simulink model "CorrienteH11"  (R2026a)
settings: Solver=FixedStepDiscrete  StopTime=1  FixedStep=1/2000  EnableMultiTasking=on
libraries: slpidlib x10
settings Model: SILPILModeSetting=veronly  ExtModeTrigDuration=10  Creator=Mutti  LastModifiedBy=Mutti
settings DataIOCC: SaveState=on  InspectSignalLogs=on
settings OptimizationCC: StrengthReduction=on  OptimizationPriority=Speed  UseRestrictQualifier=on
settings HardwareCC: ProdLargestAtomicInteger=Long  ProdLargestAtomicFloat=Double  ProdHWDeviceType=ARM Compatible->ARM Cortex-M
settings ModelReferenceCC: PropagateVarSize=During execution
settings RTWCC: SystemTargetFile=ert.tlc  GenCodeOnly=on  GenerateReport=on  BuildConfiguration=Faster Runs  IncludeHyperlinkInReport=on  LaunchReport=on  PortableWordSizes=on  CodeProfilingSaveOptions=AllData  TargetLang=C++  GenerateTraceInfo=on  GenerateTraceReport=on  GenerateTraceReportSl=on  GenerateTraceReportSf=on  GenerateTraceReportEml=on  GenerateWebview=on  GenerateCodeMetricsReport=on  GenerateCodeReplacementReport=on  Description=Embedded Coder
settings CodeAppCC: GenerateComments=off  SimulinkBlockComments=off
settings ERTTargetCC: ExtModeTransport=3.0  ExtModeStaticAllocSize=2048.0  RootIOFormat=Structure reference  TargetLangStandard=C++20 (ISO)  CodeReplacementLibrary=ARM Cortex-M  CodeInterfacePackaging=C++ class  SubcomponentCodeInterfacePackaging=C++ class  SupportNonFinite=off  SupportVariableSizeSignals=on

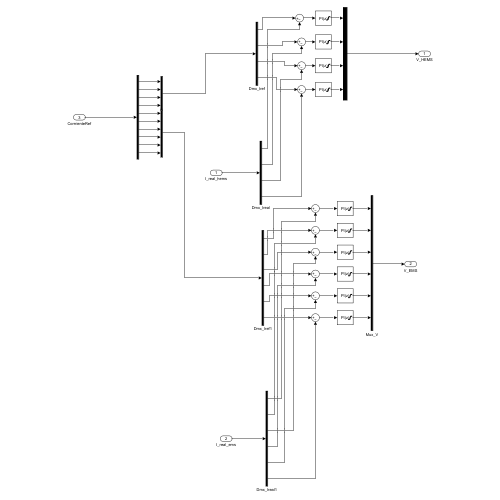
[thumbnail: Simulink's stored preview of the top-level diagram]
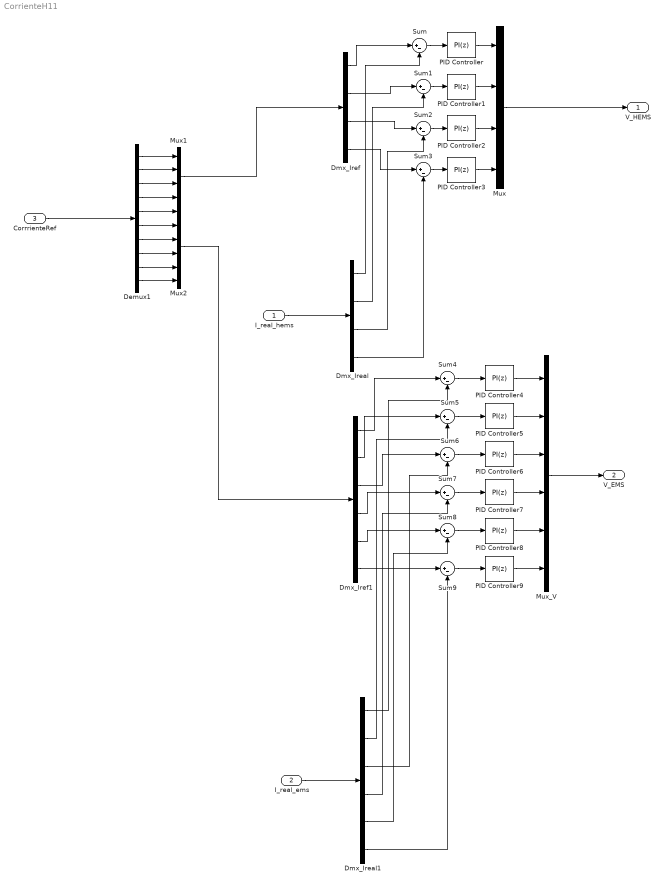
== system CorrienteH11 ==
  I_real_hems : Inport  OutDataTypeStr=double  PortDimensions=4  SampleTime=[0.00050000000000000001,0]
  I_real_ems : Inport  Port=2
  CorrrienteRef : Inport  Port=3
  Demux1 : Demux  Outputs=10
  Dmx_Ireal : Demux
  Dmx_Ireal1 : Demux  Outputs=6
  Dmx_Iref : Demux
  Dmx_Iref1 : Demux  Outputs=6
  Mux : Mux
  Mux1 : Mux
  Mux2 : Mux  Inputs=6
  Mux_V : Mux  Inputs=6
  PID Controller{,1..3} (4 alike) : slpidlib/PID Controller  Controller=PI  Form=Parallel  TimeDomain=Discrete-time  UseExternalTs=off  SampleTime=1/2000  IntegratorMethod=Trapezoidal  FilterMethod=Forward Euler  ControllerParametersSource=internal  P=4.54  I=500  UseKiTs=off  D=0  UseExternalDerivativeSource=off  N=100  UseFilter=on  TunerSelectOption=Transfer Function Based (PID Tuner App)  InitialConditionSource=internal  InitialConditionForIntegrator=0  InitialConditionForFilter=0  DifferentiatorICPrevScaledInput=0  ExternalReset=none  TrackingMode=off  Kt=1  LimitOutput=on  SatLimitsSource=internal  UpperSaturationLimit=350  LowerSaturationLimit=-350  LinearizeAsGain=on  AntiWindupMode=clamping  Kb=1  LimitIntegrator=on  UpperIntegratorSaturationLimit=350  LowerIntegratorSaturationLimit=-350  POutMin=[]  POutMax=[]  IOutMin=[]  IOutMax=[]  DOutMin=[]  DOutMax=[]  NOutMin=[]  NOutMax=[]  SumOutMin=[]  SumOutMax=[]  SaturationOutMin=[]  SaturationOutMax=[]  PParamMin=[]  PParamMax=[]  IParamMin=[]  IParamMax=[]  DParamMin=[]  DParamMax=[]  NParamMin=[]  NParamMax=[]  KbParamMin=[]  KbParamMax=[]  KtParamMin=[]  KtParamMax=[]  KbOutMin=[]  KbOutMax=[]  KtOutMin=[]  KtOutMax=[]  IntegratorOutMin=[]  IntegratorOutMax=[]  FilterOutMin=[]  FilterOutMax=[]  SumI1OutMin=[]  SumI1OutMax=[]  SumI2OutMin=[]  SumI2OutMax=[]  SumI3OutMin=[]  SumI3OutMax=[]  SumI4OutMin=[]  SumI4OutMax=[]  SumDOutMin=[]  SumDOutMax=[]  DifferentiatorOutMin=[]  DifferentiatorOutMax=[]  FilterDiffOutCoefMin=[]  FilterDiffOutCoefMax=[]  ReciprocalOutMin=[]  ReciprocalOutMax=[]  SumDenOutMin=[]  SumDenOutMax=[]  SumNumOutMin=[]  SumNumOutMax=[]  DivideOutMin=[]  DivideOutMax=[]  UdiffTsProdOutMin=[]  UdiffTsProdOutMax=[]  NTsProdOutMin=[]  NTsProdOutMax=[]  UintegralTsProdOutMin=[]  UintegralTsProdOutMax=[]  UngainTsProdOutMin=[]  UngainTsProdOutMax=[]  ClampingZeroOutDataTypeStr=Inherit: Inherit via back propagation  ClampingZeroOutMin=[]  ClampingZeroOutMax=[]  FilterDenConstantOutDataTypeStr=Inherit: Inherit via back propagation  FilterDenConstantOutMin=[]  FilterDenConstantOutMax=[]  PCopyOutDataTypeStr=Inherit: Inherit via back propagation  PCopyOutMin=[]  PCopyOutMax=[]  NCopyOutDataTypeStr=Inherit: Inherit via back propagation  NCopyOutMin=[]  NCopyOutMax=[]  IntegratorContinuousStateAttributes=''  IntegratorStateMustResolveToSignalObject=off  IntegratorRTWStateStorageClass=Auto  FilterContinuousStateAttributes=''  FilterStateMustResolveToSignalObject=off  FilterRTWStateStorageClass=Auto  ParallelPVariant=InternalParameters  IdealPVariant=Disabled  IVariant=InternalParameters  DVariant=Disabled  IntegratorVariant=Discrete  SatVariant=Enabled  AWVariant=DiscClampingParallel  PCopyVariant=Disabled  TRVariant=Disabled  FdbkBlocksVariant=Feedback  IdealPFdbkVariant=Passthrough  SatFdbkVariant=Passthrough  DerivativeFilterVariant=Disabled  NVariant=Disabled  NCopyVariant=Disabled_SignalSpec  FilterICVariant=Disabled  IntegratorICVariant=InternalICs  ExternalResetVariant=Disabled  TRSumVariant=Passthrough  SumFdbkVariant=Enabled  SumVariant=Sum_PI  TsampFilterVariant=InternalTs  TsampNgainVariant=Passthrough  TsampIntegralVariant=Disabled_SignalSpec  ExternalSaturationOutDataTypeStr=Inherit: Same as second input  DerivativeSourceVariant=Disabled  PreIntVariant=InternalPreInt
  PID Controller{4..9} (6 alike) : slpidlib/PID Controller  Controller=PI  Form=Parallel  TimeDomain=Discrete-time  UseExternalTs=off  SampleTime=1/2000  IntegratorMethod=Trapezoidal  FilterMethod=Forward Euler  ControllerParametersSource=internal  P=0.50390000000000001  I=70  UseKiTs=off  D=0  UseExternalDerivativeSource=off  N=100  UseFilter=on  TunerSelectOption=Transfer Function Based (PID Tuner App)  InitialConditionSource=internal  InitialConditionForIntegrator=0  InitialConditionForFilter=0  DifferentiatorICPrevScaledInput=0  ExternalReset=none  TrackingMode=off  Kt=1  LimitOutput=on  SatLimitsSource=internal  UpperSaturationLimit=350  LowerSaturationLimit=-350  LinearizeAsGain=on  AntiWindupMode=clamping  Kb=1  LimitIntegrator=on  UpperIntegratorSaturationLimit=350  LowerIntegratorSaturationLimit=-350  POutMin=[]  POutMax=[]  IOutMin=[]  IOutMax=[]  DOutMin=[]  DOutMax=[]  NOutMin=[]  NOutMax=[]  SumOutMin=[]  SumOutMax=[]  SaturationOutMin=[]  SaturationOutMax=[]  PParamMin=[]  PParamMax=[]  IParamMin=[]  IParamMax=[]  DParamMin=[]  DParamMax=[]  NParamMin=[]  NParamMax=[]  KbParamMin=[]  KbParamMax=[]  KtParamMin=[]  KtParamMax=[]  KbOutMin=[]  KbOutMax=[]  KtOutMin=[]  KtOutMax=[]  IntegratorOutMin=[]  IntegratorOutMax=[]  FilterOutMin=[]  FilterOutMax=[]  SumI1OutMin=[]  SumI1OutMax=[]  SumI2OutMin=[]  SumI2OutMax=[]  SumI3OutMin=[]  SumI3OutMax=[]  SumI4OutMin=[]  SumI4OutMax=[]  SumDOutMin=[]  SumDOutMax=[]  DifferentiatorOutMin=[]  DifferentiatorOutMax=[]  FilterDiffOutCoefMin=[]  FilterDiffOutCoefMax=[]  ReciprocalOutMin=[]  ReciprocalOutMax=[]  SumDenOutMin=[]  SumDenOutMax=[]  SumNumOutMin=[]  SumNumOutMax=[]  DivideOutMin=[]  DivideOutMax=[]  UdiffTsProdOutMin=[]  UdiffTsProdOutMax=[]  NTsProdOutMin=[]  NTsProdOutMax=[]  UintegralTsProdOutMin=[]  UintegralTsProdOutMax=[]  UngainTsProdOutMin=[]  UngainTsProdOutMax=[]  ClampingZeroOutDataTypeStr=Inherit: Inherit via back propagation  ClampingZeroOutMin=[]  ClampingZeroOutMax=[]  FilterDenConstantOutDataTypeStr=Inherit: Inherit via back propagation  FilterDenConstantOutMin=[]  FilterDenConstantOutMax=[]  PCopyOutDataTypeStr=Inherit: Inherit via back propagation  PCopyOutMin=[]  PCopyOutMax=[]  NCopyOutDataTypeStr=Inherit: Inherit via back propagation  NCopyOutMin=[]  NCopyOutMax=[]  IntegratorContinuousStateAttributes=''  IntegratorStateMustResolveToSignalObject=off  IntegratorRTWStateStorageClass=Auto  FilterContinuousStateAttributes=''  FilterStateMustResolveToSignalObject=off  FilterRTWStateStorageClass=Auto  ParallelPVariant=InternalParameters  IdealPVariant=Disabled  IVariant=InternalParameters  DVariant=Disabled  IntegratorVariant=Discrete  SatVariant=Enabled  AWVariant=DiscClampingParallel  PCopyVariant=Disabled  TRVariant=Disabled  FdbkBlocksVariant=Feedback  IdealPFdbkVariant=Passthrough  SatFdbkVariant=Passthrough  DerivativeFilterVariant=Disabled  NVariant=Disabled  NCopyVariant=Disabled_SignalSpec  FilterICVariant=Disabled  IntegratorICVariant=InternalICs  ExternalResetVariant=Disabled  TRSumVariant=Passthrough  SumFdbkVariant=Enabled  SumVariant=Sum_PI  TsampFilterVariant=InternalTs  TsampNgainVariant=Passthrough  TsampIntegralVariant=Disabled_SignalSpec  ExternalSaturationOutDataTypeStr=Inherit: Same as second input  DerivativeSourceVariant=Disabled  PreIntVariant=InternalPreInt
  Sum{,1..9} (10 alike) : Sum  Inputs=|+-
  V_HEMS : Outport  OutDataTypeStr=double  PortDimensions=4  SampleTime=[0.00050000000000000001,0]
  V_EMS : Outport  Port=2
  wires:
  Dmx_Iref/1 -> Sum/1
  PID Controller2/1 -> Mux/3
  Mux/1 -> V_HEMS/1
  Sum1/1 -> PID Controller1/1
  I_real_hems/1 -> Dmx_Ireal/1
  Dmx_Ireal/4 -> Sum3/2
  Dmx_Iref/3 -> Sum2/1
  Dmx_Iref/2 -> Sum1/1
  Sum/1 -> PID Controller/1
  Mux1/1 -> Dmx_Iref/1
  Dmx_Ireal/3 -> Sum2/2
  Dmx_Ireal/1 -> Sum/2
  Sum3/1 -> PID Controller3/1
  Dmx_Iref/4 -> Sum3/1
  Dmx_Ireal/2 -> Sum1/2
  PID Controller/1 -> Mux/1
  PID Controller1/1 -> Mux/2
  Sum2/1 -> PID Controller2/1
  PID Controller3/1 -> Mux/4
  Sum8/1 -> PID Controller8/1
  Mux_V/1 -> V_EMS/1
  Dmx_Iref1/6 -> Sum9/1
  Sum9/1 -> PID Controller9/1
  Dmx_Ireal1/4 -> Sum7/2
  Sum6/1 -> PID Controller6/1
  Dmx_Ireal1/3 -> Sum6/2
  Dmx_Ireal1/2 -> Sum5/2
  PID Controller5/1 -> Mux_V/2
  Sum4/1 -> PID Controller4/1
  Dmx_Ireal1/6 -> Sum9/2
  I_real_ems/1 -> Dmx_Ireal1/1
  Dmx_Iref1/1 -> Sum4/1
  Sum5/1 -> PID Controller5/1
  Dmx_Iref1/2 -> Sum5/1
  Dmx_Ireal1/5 -> Sum8/2
  Dmx_Ireal1/1 -> Sum4/2
  PID Controller7/1 -> Mux_V/4
  PID Controller9/1 -> Mux_V/6
  PID Controller6/1 -> Mux_V/3
  Dmx_Iref1/3 -> Sum6/1
  PID Controller4/1 -> Mux_V/1
  PID Controller8/1 -> Mux_V/5
  Dmx_Iref1/4 -> Sum7/1
  Sum7/1 -> PID Controller7/1
  Dmx_Iref1/5 -> Sum8/1
  Demux1/1 -> Mux1/1
  Demux1/10 -> Mux2/6
  Demux1/8 -> Mux2/4
  CorrrienteRef/1 -> Demux1/1
  Demux1/2 -> Mux1/2
  Demux1/4 -> Mux1/4
  Demux1/7 -> Mux2/3
  Demux1/9 -> Mux2/5
  Demux1/3 -> Mux1/3
  Demux1/5 -> Mux2/1
  Demux1/6 -> Mux2/2
  Mux2/1 -> Dmx_Iref1/1
